simulink model "UOIT_EV"  (R2018a)
settings: Solver=VariableStepAuto  StartTime=0.0  StopTime=1  RelTol=1e-3
model workspace (MAT data in the model file):
  AccessoryLoad = 600
  C_ref = 600
  DrCycles.C505 = [0 1 2 3 4 5 6 7 8 9 10 11 ... (1012 elements, 506x2)]
  DrCycles.FTP = [0 1 2 3 4 5 6 7 8 9 10 11 ... (4956 elements, 2478x2)]
  DrCycles.UDDS = [0 1 2 3 4 5 6 7 8 9 10 11 ... (2746 elements, 1373x2)]
  DrCycles.HWFET = [0 1 2 3 4 5 6 7 8 9 10 11 ... (1532 elements, 766x2)]
  DrCycles.US06 = [0 1 2 3 4 5 6 7 8 9 10 11 ... (1194 elements, 597x2)]
  DrCycles.US06City = [0 1 2 3 4 5 6 7 8 9 10 11 ... (466 elements, 233x2)]
  DrCycles.US06Hwy = [0 1 2 3 4 5 6 7 8 9 10 11 ... (742 elements, 371x2)]
  K = 1.04716227018
  Kc_ref = 0.12
  Ki_ref = 0.01
  Kw_ref = 1.2e-05
  MDL.MotorModel.kc = 0.0452374100719
  MDL.MotorModel.ki = 0.0166666666667
  MDL.MotorModel.kw = 5.06640055941e-05
  MDL.MotorModel.C = 628.29736211
  MDL.MotorModel.MaxTrqOut = 500
  MDL.MotorModel.MaxPwrOut = 100000
  MDL.DrivelineModel.C0 = 600
  MDL.DrivelineModel.C1 = 0.012
  MDL.DrivelineModel.C2 = 4.9e-07
  MDL.DrivelineModel.G = 3.55
  MDL.DrivelineModel.Spinloss = 6
  MDL.DrivelineModel.Ftr_max = 5000
  MDL.DriverModel.Kp = 350
  MDL.DriverModel.Ki = 0
  MDL.DriverModel.Kd = 0
  MDL.DriverModel.BrakeGain = 100
  MDL.DriverModel.Ftr_Max = 5000
  MDL.DriverModel.Ptr_Max = 100000
  MDL.BrakeSys.MaxBrakeForce = 10000
  MDL.BrakeSys.RegenFraction = 0.55
  T_max = 500
  T_ref = 300
  TimeHWFET = 765
  TimeUDDS = 1372
  TimeUS06 = 596
  aeroDragCoeff = 0.38
  airDensity = 1.23
  energyCapacity = 12.6
  frontArea = 2.1
  gravity = 9.81
  inclinationAngle = 0
  inertialMassVeh = 2392
  initialSOC = 0.95
  internalResistance = 0.1
  massVeh = 2300
  openCircuitVoltage = 340
  rollingResistCoeff = 0.01
  w_max = 524
  w_ref = 834
  wheelRadius = 0.34
libraries: autolibmotorctrlr x4, simulink x3
(part 1 of 3)
settings Model: Creator=100655384  LastModifiedBy=100655384

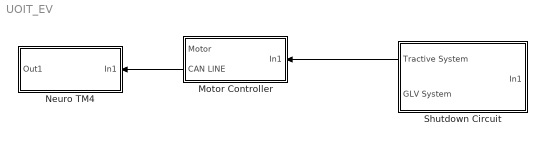
== system UOIT_EV ==
  Motor Controller : Subsystem
  Neuro TM4 : Subsystem
  Shutdown Circuit : Subsystem
  wires:
  Shutdown Circuit/1(Tractive System) -> Motor Controller/1(In1)
  Motor Controller/2(CAN LINE) -> Neuro TM4/1(In1)
